simulink model "transfer_1"  (R2022a)
settings: Solver=VariableStepAuto  StartTime=0.0  StopTime=10.0  RelTol=1e-3
settings Model: Creator=olya-  LastModifiedBy=novik
settings ModelReferenceCC: EnableRefExpFcnMdlSchedulingChecks=off
settings RTWCC: Description=Generic Real-Time Target

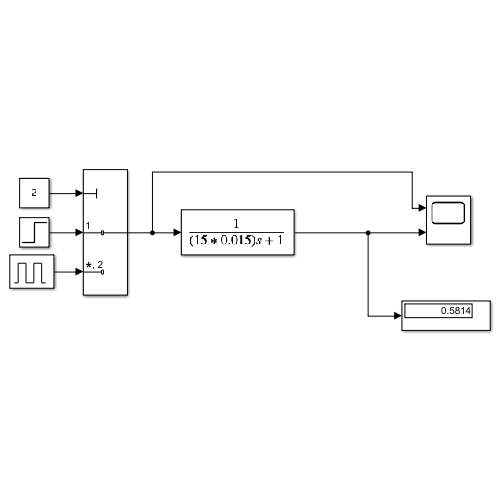
[thumbnail: Simulink's stored preview of the top-level diagram]
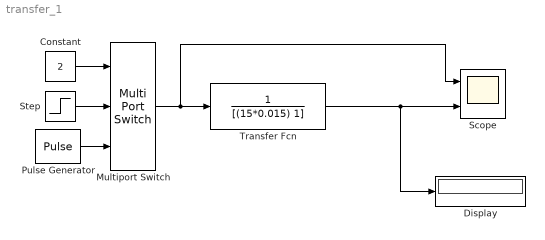
== system transfer_1 ==
  Constant : Constant  Value=2
  Display : Display
  Multiport Switch : MultiPortSwitch  Inputs=2  SaturateOnIntegerOverflow=off  InputSameDT=off
  Pulse Generator : DiscretePulseGenerator  PulseType=Time based  Amplitude=50  PulseWidth=50
  Scope : Scope  NumInputPorts=2
  Step : Step  After=50  SampleTime=0
  Transfer Fcn : TransferFcn  Denominator=[(15*0.015) 1]
  wires:
  Transfer Fcn/1 -> Display/1, Scope/2
  Multiport Switch/1 -> Transfer Fcn/1, Scope/1
  Step/1 -> Multiport Switch/2
  Pulse Generator/1 -> Multiport Switch/3
  Constant/1 -> Multiport Switch/1
